simulink model "redundancy"  (R2013b)
settings: Solver=FixedStepDiscrete  SolverMode=SingleTasking  StartTime=0  StopTime=8000  RelTol=1e-3
model workspace (MAT data in the model file):
  logicAddr = 2
settings Model: Creator=qiji  LastModifiedBy=qiji
settings DataIOCC: SaveOutput=off  SaveTime=off
settings OptimizationCC: BlockReduction=off  ConditionallyExecuteInputs=off  InlineParams=on
settings DebuggingCC: UnderspecifiedInitializationDetection=Simplified  MultiTaskDSMMsg=warning  MultiTaskCondExecSysMsg=none  SingleTaskRateTransMsg=error  SFUnusedDataAndEventsDiag=none
settings RTWCC: IncludeERTFirstTime=on
settings GRTTargetCC: CodeReplacementLibrary=None  CPPClassGenCompliant=on
settings ConfigurationSet: Description=SimMechanics 2G

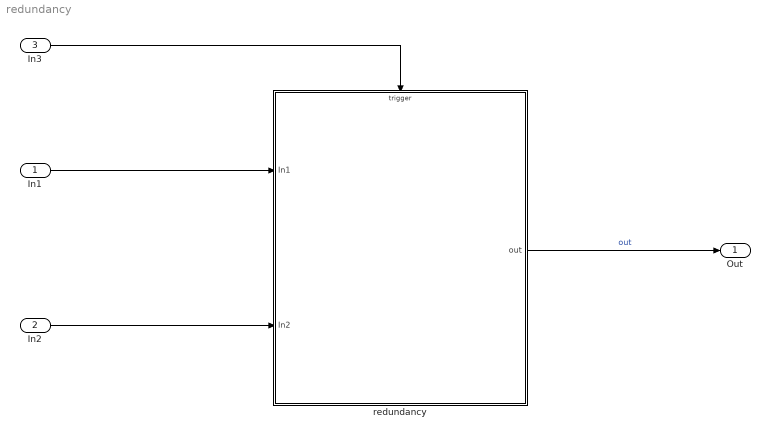
== system redundancy ==
  In1 : Inport  OutDataTypeStr=uint32  PortDimensions=1  SampleTime=[1,0]
  In2 : Inport  Port=2  OutDataTypeStr=uint32  PortDimensions=1  SampleTime=[1,0]
  In3 : Inport  Port=3  OutDataTypeStr=boolean  PortDimensions=1  SampleTime=[1,0]
  redundancy : Stateflow chart  TreatAsAtomicUnit=on
  Out : Outport  OutDataTypeStr=uint32  PortDimensions=1  SampleTime=[1,0]
  wires:
  In3/1 -> redundancy/Trigger
  In1/1 -> redundancy/1(In1)
  In2/1 -> redundancy/2(In2)
  redundancy/1(out) -> Out/1  "out"

== stateflow chart redundancy/redundancy ==
  settings: executeAtInitialization=1  initializeOutput=1
  state sign_maker [parallel]
    settings: executionOrder=1
    state sign1 [parallel]
      settings: executionOrder=1
      state trans
        sign_maker.sign1.trans -> sign_maker.sign1.trans [order 1] : CLK
            | {
            | buffer = bitoperate.shiftbit(buffer, 1) + In1;
            | count++;
            | }
      state none
        en:
        count=2;
        buffer=1;
      state judge
      (default) -> sign_maker.sign1.none : {count=0;buffer=0;}
      sign_maker.sign1.none -> sign_maker.sign1.trans : [In1==1]{sign1 = true;}
      sign_maker.sign1.judge -> sign_maker.sign1.trans [order 2] : {buffer=0;count=0;}
      sign_maker.sign1.judge -> sign_maker.sign1.none [order 1] : [judgeEnd(buffer)]
          | {sign1 = false;}
      sign_maker.sign1.trans -> sign_maker.sign1.judge [order 1] : [count==32]
          | {buffer=ManchesterDecoding(buffer);
          | }
    state sign2 [parallel]
      settings: executionOrder=2
      state trans
        sign_maker.sign2.trans -> sign_maker.sign2.trans [order 1] : CLK
            | {
            | buffer = bitoperate.shiftbit(buffer, 1) + In2;
            | count++;
            | }
      state none
        en:
        count=2;
        buffer=1;
      state judge
      (default) -> sign_maker.sign2.none : {count=0;buffer=0;}
      sign_maker.sign2.none -> sign_maker.sign2.trans : [In2==1]{sign2 = true;}
      sign_maker.sign2.judge -> sign_maker.sign2.trans [order 2] : {buffer=0;count=0;}
      sign_maker.sign2.judge -> sign_maker.sign2.none [order 1] : [judgeEnd(buffer)]
          | {sign2 = false;}
      sign_maker.sign2.trans -> sign_maker.sign2.judge [order 1] : [count==32]
          | {buffer=ManchesterDecoding(buffer);
          | }
  state bitoperate [group]
  note: 从上一个接收事件后总线寂静1.4ms则产生一总线寂静的通知
  state Timer1 [parallel]
    settings: executionOrder=2
    state Timer
    state start
    state TimeOut
      entry:
      trust = false;
    start -> Timer : [judge(sign1, sign2, trust) == false]
    (default) -> start
    Timer -> start [order 1] : [judge(sign1, sign2,  trust) == true]
    TimeOut -> start
    Timer -> TimeOut [order 2] : [after(140, CLK) && judge(sign1, sign2,  trust) == false]
  note: 上一个主帧接收后1.3ms没有收到主帧产生一个主帧超时的通知。
  note: 收到主帧后42.7us没有收到从帧产生从帧超时的通知。
  note: 信任线未收到数据，而观察线收到数据时切换
  state observer [parallel]
    settings: executionOrder=3
    state A
      entry:
      trust = true;
    state B
      entry:
      trust = false;
    observer.A -> observer.B : [judge(sign1, sign2, trust) == false]
    (default) -> observer.A
    observer.B -> observer.A : [judge(sign1, sign2, trust) == false]
  state trans [parallel]
    settings: executionOrder=4
    state A
      during:
      out = In1;
    state B
      during:
      out = In2;
    trans.A -> trans.B : [trust == false]{out = In2;}
    (default) -> trans.A
    trans.B -> trans.A : [trust == true]{out = In1;}
  data: r function_output boolean; data function_input uint16; buffer local uint32; count local uint32; buffer local uint32; count local uint32; r function_output uint32; data function_input uint32; num function_input uint32; r function_output uint32; data function_input uint32; num function_input uint32; r function_output uint32; r function_output boolean; dataIn1 function_input uint32; dataIn2 function_input uint32; t function_input boolean; r function_output boolean; dataIn1 function_input boolean; dataIn2 function_input boolean; t function_input boolean; In1 input uint32; In2 input uint32; out output uint32; trust local boolean =true; sign1 local boolean; sign2 local boolean
  events: CLK input RISING_EDGE_EVENT
  function r = judgeEnd(data):
    | function r = judgeEnd(data)
    | bit1 = bitget(data, 1);
    | bit2 = bitget(data, 2);
    | bit3 = bitget(data, 3);
    | bit4 = bitget(data, 4);
    | if bit1==1 && bit2==1 && bit3==0 && bit4==0
    |     r = true;
    | else
    |     r = false;
    | end
  function r = ManchesterDecoding(data):
    | function r = ManchesterDecoding(data)
    | r = uint32(0);
    | for i = (1:2:32)
    |     x0 = bitget(data, i);
    |     x1 = bitget(data, i+1);
    |     if x0==0 && x1==1
    |         r = bitset(r, (i+1)/2, 1);
    |     else
    |         r = bitset(r, (i+1)/2, 0);
    |     end
    | end
  function r = getbit(num):
    | function r = getbit(num)
    | r = bitget(num, 32);
  function r = shiftbit(data, num):
    | function r = shiftbit(data, num)
    | r = bitshift(data, num);
    | %for i=1:cnt
    | %   r = bitset(r, i, 0);
    | %end
  function r = judge(dataIn1, dataIn2, t):
    | function r = judge(dataIn1, dataIn2, t)
    | r = true;
    | if t == true
    |     if dataIn1==false
    |         r = false;
    |     end
    | else
    |     if dataIn2==false
    |         r = false;
    |     end
    | end
  function r = judge( dataIn1, dataIn2, t):
    | function r = judge( dataIn1, dataIn2, t)
    | r = true;
    | % 如果数据线1没有收到数据而数据线2收到了
    | if t == true
    |     if dataIn1==false && dataIn2==true
    |         r = false;
    |     end
    | else
    |     if dataIn2==false && dataIn1==true
    |         r = false;
    |     end
    | end
